simulink model "et_robocon"  (R2014b)
settings: Solver=ode3  SolverMode=SingleTasking  StartTime=0.0  StopTime=10.0  RelTol=1e-3
undefined symbols (not defined in the file): balancerStates_Bus0, Batt, current_mode_status, current_task_operation_status, GYRO, Init_Bus0, K, lightCalib, PHI, R, RM, TRACK_MODE_LIST, W
libraries: legonxtlib x23, ControllersFcns x5, simulink_extras x4, NXTFcns x2, simulink x2, gyro_calibration_algorithm_atomic_sub_chart_library x1, light_sensor_calibration_algorithm_atomic_sub_chart_library x1, plantNXT x1
(part 2 of 2)

== stateflow chart et_robocon/Main Controller/normal_operation_modes.line_following ==
  state see_saw_mode
    entry:
    des_vel = single(0.0);
    desired_tail = single(0.0);
    BT_status_out = single(11);
    Speak;
    during:
    normalizedLight = processLight(sensors.light,lightCalib);
    PWM.tail = tail_controller(sensors.theta_T, desired_tail);
    state Waiting
      during:
      StatusLCD(uint16(300));
    state light = processLight(rawLight,lightCalib) [function]
    state cmd = balance_ctrl(balancerStates,desired_velocity,battery) [function]
    state StandUp
      entry:
      StatusLCD(uint16(301));
      initFlags.theta = single(1);
      initFlags.gyroReset = single(1);
    state cmd = lineTracker(desiredLight,light,trackingPower,battery) [function]
    state Balancing
      state SeesawLogic [parallel]
        settings: executionOrder=2
        state MoveForwardSlowly
          entry:
          StatusLCD(uint16(302));
          initFlags.theta = single(0);
          initFlags.gyroReset = single(0);
          des_vel = single(0.0005);
          %desired_states = balancerStates_Bus0;
          %turningPWM = single(0);
        state BridgeTest [commented out]
          entry:
          Speak;
          StatusLCD(uint16(3001));
          des_vel = single(0.0);
          desired_phi = states.phi;
          during:
          des_vel = single(0.03);
          turningPWM = phiController(desired_phi,states.phi,sensors.battery);
        state StationnaryBalance
          entry:
          Speak;
          StatusLCD(uint16(303));
          %StatusLCD(uint16(single(0.15)));
          des_vel = single(0.0005);
          desired_phi = states.phi;
          exit:
          turningPWM =     phiController(desired_phi,states.phi,sensors.battery);
          %lineTracker(single(-0.1), normalizedLight, single(1.3), sensors.battery);
        state Curvature
          entry:
          Speak;
          Speak;
          Speak;
          %StatusLCD(uint16(305));
          state Slowdown
            entry:
            des_vel =single(0.2);
            during:
            des_vel = des_vel-single(0.0005);
            turningPWM = lineTracker(single(-0.1), normalizedLight, single(0.8), sensors.battery);
          state Const
            during:
            turningPWM = lineTracker(single(-0.1), normalizedLight, single(1.2), sensors.battery);
          (default) -> Slowdown
          Slowdown -> Const : [des_vel<=0.09]
        state SpeedUp
          entry:
          Speak;
          StatusLCD(uint16(304));
          %des_vel = single(0.001);
          during:
          des_vel = des_vel+single(0.0005);
          turningPWM = lineTracker(single(-0.15), normalizedLight, single(1.2), sensors.battery);
        state ConstantSpeed
          entry:
          Speak;
          StatusLCD(uint16(305));
          during:
          turningPWM = lineTracker(single(-0.15), normalizedLight, single(1.2), sensors.battery);
        state Ramp
          state RampUpOne
            entry:
            desired_phi = states.phi;
            storedphi = states.phi;
            Speak;
            StatusLCD(uint16(3061));
            des_vel = single(0.05);
            during:
            turningPWM = lineTracker(single(-0.1),normalizedLight,single(0.5),sensors.battery)+...
            phiController(desired_phi,states.phi,sensors.battery);
            %storedphi = states.phi;
          state BridgeTest
            entry:
            Speak;
            Speak;
            StatusLCD(uint16(3062));
            des_vel = single(0.04);
            desired_phi = storedphi;
            during:
            %des_vel = single(0.04);
            turningPWM = phiController(desired_phi,states.phi,sensors.battery);
          state RampUpTwo
            entry:
            desired_phi = states.phi;
            Speak;
            StatusLCD(uint16(3063));
            des_vel = single(0.04);
            during:
            turningPWM = lineTracker(single(-0.1),normalizedLight,single(0.5),sensors.battery)+...
            phiController(desired_phi,states.phi,sensors.battery);
          state SlowtoRotate
            entry: StatusLCD(uint16(3064));
            Speak;
            des_vel = single(0.03);
            desired_phi = states.phi;
            during:
            des_vel = des_vel-single(0.01);
            turningPWM = phiController(desired_phi,states.phi,sensors.battery);
          state Stop
            entry: StatusLCD(uint16(3065));
            des_vel = single(0.0);
            desired_phi = states.phi;
            during:
            turningPWM = phiController(desired_phi,states.phi,sensors.battery);
          state RotateInPlace [commented out]
            entry: StatusLCD(uint16(3065));
            des_vel = single(0.0);
            desiredangle = states.phi+single(180.0);
            desired_phi = states.phi+single(0.5);
            during:
            %desired_phi = desired_phi+10.0;
            %des_vel = single(0.07);
            turningPWM = phiController(desired_phi,states.phi,sensors.battery);
            desired_phi = desired_phi+single(0.5);
          (default) -> RampUpOne
          RampUpOne -> see_saw_mode.Balancing.SeesawLogic.Ramp.BridgeTest : [after(2,sec) && states.balancerStates.psi_dot<single(-0.8) && states.balancerStates.theta_dot>single(2.8)]
          see_saw_mode.Balancing.SeesawLogic.Ramp.BridgeTest -> RampUpTwo : [(after(2,sec) && states.balancerStates.theta_dot<- single(3)) || sensors.touch]
          RampUpTwo -> SlowtoRotate : [after(1,sec)]
          SlowtoRotate -> Stop : [des_vel<=0.01]
          SlowtoRotate -> RotateInPlace [commented out] : [des_vel<=0.01]
          RotateInPlace -> Stop [commented out] : [states.phi>=desiredangle]
        state ApproachtoRamp_1 [commented out]
          entry:
          desired_phi = states.phi;
          Speak;
          StatusLCD(uint16(304));
          des_vel = single(0.1);
          during:
          turningPWM = lineTracker(single(-0.1),normalizedLight,single(0.0),sensors.battery)+...
          phiController(desired_phi,states.phi,sensors.battery);
        state testthetadot [commented out]
          entry:
          Speak;
          StatusLCD(uint16(1000));
          during:
          turningPWM = single(0);
          StatusLCD(uint16(states.balancerStates.theta_dot));
        state ApproachToSeeSaw [commented out]
          entry: %debugFlag = uint16(604);
          during:
          turningPWM = phiController(states.phi,desired_phi, sensors.battery);
          exit:
          turningPWM = single(0);
        state Seesaw [commented out]
          state ControlledGoingUp [commented out]
            entry:
            phi0 = states.phi;
            desired_phi = phi0;
            exit: turningPWM = single(0);
            state JumpOnIt [commented out]
              entry:
              Speak;
              debugFlag = uint16(606);
              theta_ref = states.balancerStates.theta;
              des_vel = single(0.15);
              du: turningPWM = phiController(states.phi,desired_phi, sensors.battery);
            state GoingUP [commented out]
              entry:
              debugFlag = uint16(607);
              des_vel = single(0.1);
              during:
              turningPWM = phiController(states.phi,desired_phi, sensors.battery)+...
              single(3)*lineTracker(single(0.15), normalizedLight, single(1), sensors.battery);
              exit:
              des_vel = single(0);
            state WaitForPrincess [commented out]
              entry:
              debugFlag = uint16(608);
              BT_status_out = single(12);
              Speak;
              du:
              turningPWM = phiController(states.phi,desired_phi,sensors.battery);
            (default) -> JumpOnIt [commented out]
            JumpOnIt -> GoingUP [commented out] : [states.balancerStates.theta >= theta_ref+single(1.6)]
            GoingUP -> WaitForPrincess [commented out] : [states.balancerStates.theta >= theta_ref + single(18)]
          state GoingDown [commented out]
            during:
            turningPWM = single(-1.3)*lineTracker(single(0.7), normalizedLight, single(1.2), sensors.battery)+...
            single(1)*phiController(states.phi,desired_phi,sensors.battery);
            state GoingBack [commented out]
              entry:
              debugFlag = uint16(609);
              des_vel = single(-0.06);
              exit:
              des_vel = single(-0.06);
            state WaitForPrincess2 [commented out]
              entry:
              debugFlag = uint16(610);
              BT_status_out = single(16);
              Speak;
              %during:turningPWM = phiController(states.phi,desired_phi,sensors.battery);
            state GetOff [commented out]
              entry:
              debugFlag = uint16(611);
              des_vel = single(-0.1);
            (default) -> GoingBack [commented out]
            GoingBack -> WaitForPrincess2 [commented out] : [states.balancerStates.theta <= theta_ref + single(15)]
            WaitForPrincess2 -> GetOff [commented out] : [sensors.BT_status_in == single(21)]{Speak;}
          state GetOff1 [commented out]
            entry:
            debugFlag = uint16(6112);
            des_vel = single(-0.08);
            du:
            turningPWM = phiController(states.phi,desired_phi+single(0.05),sensors.battery);
          state FindingLine [commented out]
            en:
            turningPWM = phiController(states.phi,desired_phi,sensors.battery);
            des_vel = single(0);
            state TurnAndBackup [commented out]
              entry:
              debugFlag = uint16(612);
              BT_status_out = single(14);
              Speak;
              du:
              desired_phi = desired_phi - single(0.003);
              des_vel = single(0);
              turningPWM = phiController(states.phi,desired_phi,sensors.battery);
            state HuntLine [commented out]
              entry: debugFlag = uint16(613)
              desired_phi = states.phi;
              theta_ref_2 = states.balancerStates.theta;
              du: turningPWM = phiController(states.phi,desired_phi,sensors.battery);
              state GoForward [commented out]
                en:  des_vel= single(0.04);
                entry: debugFlag = uint16(6131);
              state BackUpB [commented out]
                en: des_vel = single(-0.04)
                entry: debugFlag = uint16(6132);
              BackUpB -> GoForward [commented out] : [states.balancerStates.theta <= theta_ref_2 - single(3) ]
              (default) -> BackUpB [commented out]
              GoForward -> BackUpB [commented out] : [states.balancerStates.theta >= theta_ref_2 + single(3) ]
            state TurnAndBackup1 [commented out]
              entry:
              Speak
              debugFlag = uint16(614);
              des_vel = des_vel / single(3);
              du:
              desired_phi = desired_phi - single(0.003);
              turningPWM = phiController(states.phi,desired_phi,sensors.battery);
            state GoForwardUntilLine [commented out]
              en:
              Speak;
              debugFlag = uint16(615)
              des_vel = single(0);
            (default) -> TurnAndBackup [commented out]
            TurnAndBackup -> HuntLine [commented out] : [phi0-states.phi > single(1.6)]
            HuntLine -> TurnAndBackup1 [commented out] : [normalizedLight >= single(0.5)]
            TurnAndBackup1 -> GoForwardUntilLine [commented out] : [phi0-states.phi > single(2.3)]
          (default) -> ControlledGoingUp [commented out]
          WaitForPrincess -> GoingDown [commented out] : [sensors.BT_status_in == single(20)]{Speak;}
          GoingDown -> GetOff1 [commented out] : [states.balancerStates.theta <= theta_ref ]
          GetOff1 -> FindingLine [commented out] : [states.balancerStates.theta <= theta_ref - single(5)]
        state RaceDone [commented out]
          entry: debugFlag = uint16(599);
          BT_status_out = single(15);
          Speak;
          current_mode_status = OperationModeStatusEnum.SUCCESSFULLY_COMPLETED;
        (default) -> MoveForwardSlowly
        MoveForwardSlowly -> StationnaryBalance : after(2,sec)
        ApproachtoRamp_1 -> see_saw_mode.Balancing.SeesawLogic.BridgeTest [commented out] : [sensors.touch]
        StationnaryBalance -> SpeedUp : after(0.08,sec)
        Curvature -> SpeedUp : [states.phi<15 && -15<states.phi]
        SpeedUp -> ConstantSpeed : [des_vel>=0.15]
        ConstantSpeed -> Curvature [order 1] : [ (30 <states.phi || states.phi<-30) && 1 == 0]
        ConstantSpeed -> Ramp [order 2] : [sensors.touch || states.balancerStates.theta_dot<single(0.8)]
        ConstantSpeed -> testthetadot [commented out] : [sensors.touch]
        ConstantSpeed -> ApproachtoRamp_1 [commented out] : [sensors.touch || states.balancerStates.theta_dot<single(0.7)]
        ApproachToSeeSaw -> Seesaw [commented out] : [states.balancerStates.theta_dot < single(1)]
        GoForwardUntilLine -> RaceDone [commented out] : after(1,sec)
      state After [parallel]
        during:
        forwardPWM = balance_ctrl(states.balancerStates, des_vel ,sensors.battery)
        PWM.left = forwardPWM + turningPWM;
        PWM.right = forwardPWM - turningPWM;
        settings: executionOrder=1
    (default) -> Waiting
    Waiting -> StandUp : [sensors.touch]
    StandUp -> Balancing
  data: rawLight function_input single size=1; lightCalib function_input Bus: Light_Bus size=1; light function_output; balancerStates function_input Bus: Balancer_States_Bus size=1; desired_velocity function_input single size=1; battery function_input double size=1; cmd function_output single size=1; cmd function_output single size=1; desiredLight function_input single size=1; light function_input single size=1; trackingPower function_input single size=1; battery function_input double size=1; sensors input Bus: Sensors_Bus size=1; lightCalib data_store_memory; current_task_operation_status data_store_memory; PWM output Bus: PWM_bus size=1; initFlags output Bus: Init_Bus size=1; desired_tail local; balancerStates_Bus0 parameter; turningPWM local; states input; BT_status_out output; normalizedLight local; forwardPWM local; des_vel local; desired_phi local; desiredangle local; storedphi local
